simulink model "Events5"  (Simulink 8.7)
settings: Solver=FixedStepDiscrete  StartTime=0.0  StopTime=inf  RelTol=1e-3
settings Model: Creator=scaife  LastModifiedBy=hamza  ExtModeAutoUpdateStatusClock=off
settings DataIOCC: SignalLoggingSaveFormat=ModelDataLogs  SignalLoggingName=sigsOut
settings OptimizationCC: InitFltsAndDblsToZero=on
settings DebuggingCC: AlgebraicLoopMsg=error  SaveWithParameterizedLinksMsg=none  SignalResolutionControl=TryResolveAllWithWarning  MultiTaskDSMMsg=warning  MultiTaskCondExecSysMsg=none
settings HardwareCC: TargetUnknown=on
settings SFSimCC: SimParseCustomCode=off
settings GRTTargetCC: TargetFcnLib=ansi_tfl_tmw.mat  ModelReferenceCompliant=off  ParMdlRefBuildCompliant=off  CompOptLevelCompliant=off  ConcurrentExecutionCompliant=off  GeneratePreprocessorConditionals=Use local settings  CombineOutputUpdateFcns=off  MatFileLogging=off  MATLABClassNameForMDSCustomization=Simulink.SoftwareTarget.TargetSpecificTriggerConfigurationBase  GRTInterface=on

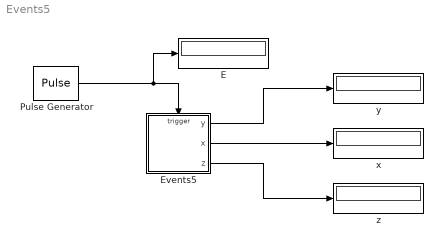
== system Events5 ==
  E : Display
  Events5 : Stateflow chart  TreatAsAtomicUnit=on
  Pulse Generator : DiscretePulseGenerator
  x : Display
  y : Display
  z : Display
  wires:
  Events5/2(x) -> x/1
  Events5/3(z) -> z/1
  Events5/1(y) -> y/1
  Pulse Generator/1 -> E/1, Events5/Trigger

== stateflow chart Events5 ==
  state Top1 [parallel]
    settings: executionOrder=1
    state A/
      en: y++
    state D/
      en: y++
    state E/
      en: y++
    (default) -> A
    E -> A : E/F;z++
    A -> D : E/send(F,Top2);z++
    D -> E : E/send(F,Top2);z++
  state Top2 [parallel]
    settings: executionOrder=2
    state B/
      en: x++
    state C/
      en: x++
    (default) -> B
    C -> B : F
    B -> C : F
  data: y output double; x output double; z output double
  events: E input EITHER_EDGE_EVENT; F local EITHER_EDGE_EVENT
